simulink model "vehicle_6dof_model"  (R2025b)
settings: Solver=VariableStepAuto  StartTime=0.0  StopTime=30.0  RelTol=1e-3
model workspace (MAT data in the model file):
  mmoi = [0.01211163  -3.59e-06  1.486e-05; -3.59e-06  0.01211098  -4.75e-07; 1.486e-05  -4.75e-07  0.00012254]
libraries: aerolibanim x1, aerolibanimutils x1
settings Model: Creator=Josh Fernandez  LastModifiedBy=Gumpp

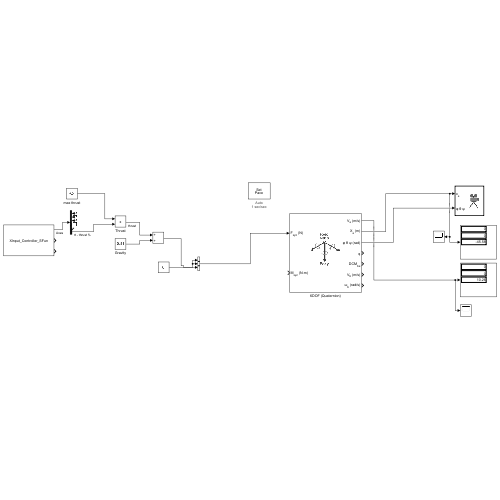
[thumbnail: Simulink's stored preview of the top-level diagram]
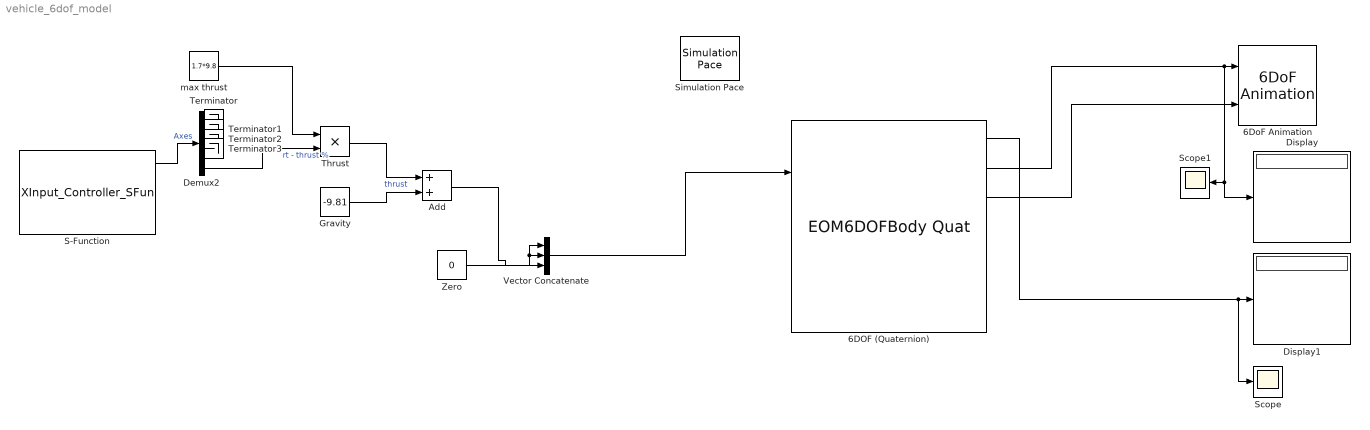
== system vehicle_6dof_model ==
  6DOF (Quaternion) : EOM6DOFBodyQuat  mass_0=.5384  inertia=mmoi
  6DoF Animation : aerolibanim/6DoF Animation  u1=[0 4000 -2000 2000 -5000 -3000]  u2=0.1  u3=1.0  u4=[4000 0 -5000]  u5=Fixed position  u6=[2000 500 -3150]  u7=10  u8=on
  Add : Sum
  Demux2 : Demux  Outputs=6
  Display : Display
  Display1 : Display
  Gravity : Constant  Value=-9.81
  S-Function : S-Function  FunctionName=XInput_Controller_SFun  Parameters=1  SFunctionDeploymentMode=off  EnableBusSupport=off
  Scope : Scope
      settings: ActiveDisplayYMinimum=-77.563316542972075  ActiveDisplayYMaximum=42.126312482587238
  Scope1 : Scope
      settings: ActiveDisplayYMinimum=-323.6001599308525  ActiveDisplayYMaximum=35.955573325650271
  Simulation Pace : aerolibanimutils/Simulation Pace  SimulationPace=1  SleepMode=Auto  OutputPaceError=off  SampleTime=1/30
  Terminator{,1..3} (4 alike) : Terminator
  Thrust : Product
  Vector Concatenate : Concatenate  NumInputs=3
  Zero : Constant  Value=0  OutDataTypeStr=Inherit: Inherit via back propagation
  max thrust : Constant  Value=1.7*9.8
  wires:
  6DOF (Quaternion)/2 -> Scope1/1, Display/1, 6DoF Animation/1
  6DOF (Quaternion)/3 -> 6DoF Animation/2
  S-Function/1 -> Demux2/1  "Axes"
  Zero/1 -> Vector Concatenate/1, Vector Concatenate/2
  Vector Concatenate/1 -> 6DOF (Quaternion)/1
  Demux2/1 -> Terminator/1
  Demux2/6 -> Thrust/2  "rt - thrust %"
  max thrust/1 -> Thrust/1
  Demux2/2 -> Terminator1/1
  Demux2/3 -> Terminator2/1
  Add/1 -> Vector Concatenate/3
  Thrust/1 -> Add/1  "thrust"
  Gravity/1 -> Add/2
  6DOF (Quaternion)/1 -> Scope/1, Display1/1
